simulink model "QUESTION1A"  (R2021b)
settings: Solver=VariableStepAuto  StartTime=0.0  StopTime=10.0  RelTol=1e-3
settings Model: Creator=Progg  LastModifiedBy=Progg

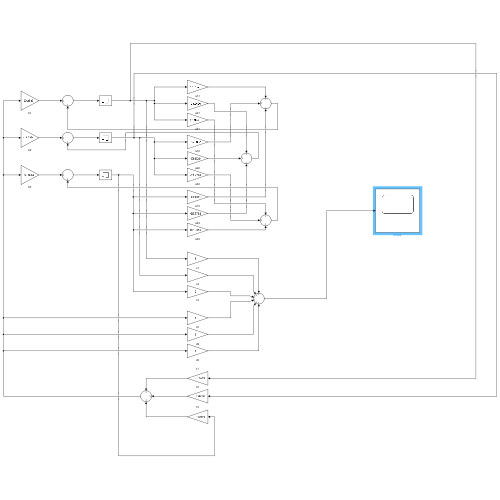
[thumbnail: Simulink's stored preview of the top-level diagram]
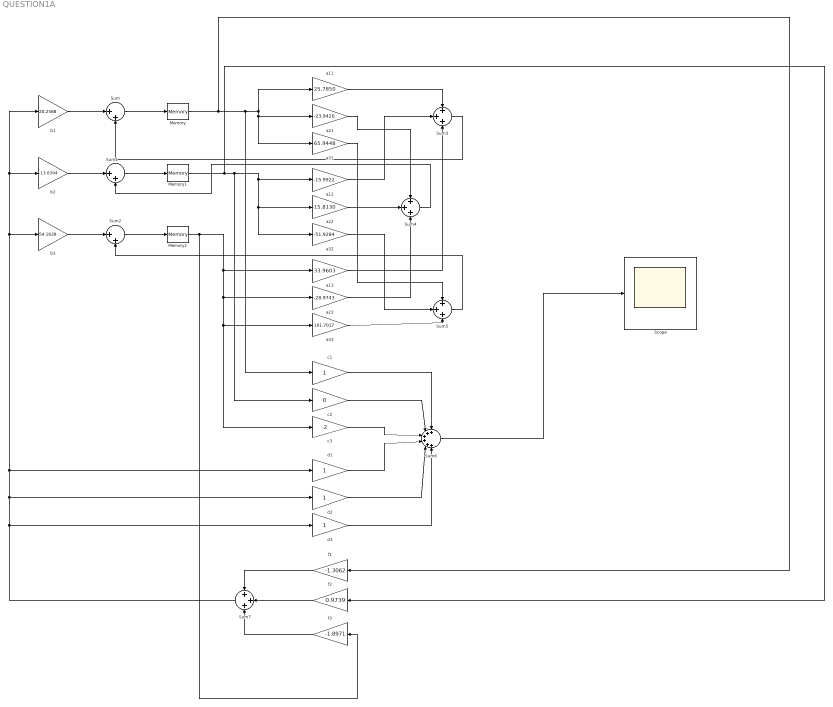
== system QUESTION1A ==
  Memory : Memory  InitialCondition=5
  Memory1 : Memory  InitialCondition=5
  Memory2 : Memory  InitialCondition=5
  Scope : Scope
  Sum : Sum  Inputs=|++
  Sum1 : Sum  Inputs=|++
  Sum2 : Sum  Inputs=|++
  Sum{3..5,7} (4 alike) : Sum  Inputs=+++
  Sum6 : Sum  Inputs=++++++
  a11 : Gain  Gain=25.7850
  a12 : Gain  Gain=-15.9922
  a13 : Gain  Gain=33.9603
  a21 : Gain  Gain=-23.9420
  a22 : Gain  Gain=15.8130
  a23 : Gain  Gain=-28.9743
  a31 : Gain  Gain=65.9448
  a32 : Gain  Gain=-51.9284
  a33 : Gain  Gain=101.7017
  b1 : Gain  Gain=20.2588
  b2 : Gain  Gain=-13.6394
  b3 : Gain  Gain=54.1639
  c1 : Gain
  c2 : Gain  Gain=0
  c3 : Gain  Gain=-2
  d1 : Gain
  d2 : Gain
  d3 : Gain
  f1 : Gain  Gain=-1.3062
  f2 : Gain  Gain=0.9739
  f3 : Gain  Gain=-1.8971
  wires:
  a32/1 -> Sum5/2
  c2/1 -> Sum6/2
  Sum2/1 -> Memory2/1
  b1/1 -> Sum/1
  Sum5/1 -> Sum2/2
  a23/1 -> Sum4/3
  a11/1 -> Sum3/1
  a22/1 -> Sum4/2
  b3/1 -> Sum2/1
  a31/1 -> Sum5/1
  Sum7/1 -> b1/1, b2/1, b3/1, d1/1, d2/1, d3/1
  Sum4/1 -> Sum1/2
  a12/1 -> Sum3/2
  a33/1 -> Sum5/3
  b2/1 -> Sum1/1
  a13/1 -> Sum3/3
  Sum/1 -> Memory/1
  a21/1 -> Sum4/1
  d1/1 -> Sum6/4
  d3/1 -> Sum6/6
  Sum1/1 -> Memory1/1
  d2/1 -> Sum6/5
  Sum3/1 -> Sum/2
  Sum6/1 -> Scope/1
  c1/1 -> Sum6/1
  c3/1 -> Sum6/3
  f2/1 -> Sum7/2
  f1/1 -> Sum7/1
  f3/1 -> Sum7/3
  Memory/1 -> c1/1, a31/1, a21/1, a11/1, f1/1
  Memory1/1 -> f2/1, c2/1, a32/1, a22/1, a12/1
  Memory2/1 -> c3/1, a33/1, a23/1, a13/1, f3/1
